simulink library "carnotUIBK"  (R2018b)
settings: Solver=VariableStepAuto  StartTime=0.0  StopTime=10.0  RelTol=1e-3  EnableMultiTasking=on
values from neighbouring files (symbols this model uses):
  A = 7*10*2    (= 140)    [theta_ground_v1.m]    (also in xlswrite1.m = num2cell(data))
  amb_factor = 1    [DOOR.m]    (also in WALL.m; WINDOW.m = 0)
  area = obj.width * obj.height    [DOOR.m]    (also in RES.m = []; ROOM.m = 0; THERMALZONE.m = area + room(kk).area; WALL.m = area - obj.doors(jj).calc_area())
  B = A/(0.5 * P)    (= 8.23529411765)    [theta_ground_v1.m]
  boundary = BOUNDARY()    [BUILDING.m]    (also in WALL.m = '')
  building = obj    [BUILDING.m]    (also in create_building_automatic.m = building.save(); ini_building_automatic.m = building.add_variant_hvac(building.variant_hvac, hvac); load_building_automatic.m = building.save())
  C = zeros(1,length(d)+1)    [CONSTRUCTION.m]    (also in DOOR.m = [0 0 0]; WALL.m = [0 0 0]; WINDOW.m = [0 0 0])
  control = 2    [GAIN.m]    (also in GAINS.m)
  cp = str2num(value)    [CONSTRUCTION.m]
  height = 0    [DOOR.m]    (also in ROOM.m; THERMALZONE.m; WALL.m; WINDOW.m)
  p = [timevec_weather weather(:,12)]    [BOUNDARY.m]    (also in WEATHER.m = 0; init_carnotUIBK.m = cell2mat(carnotUIBKpaths(i,2)))
  rho = str2num(value)    [CONSTRUCTION.m]    (also in theta_ground_v1.m = 2000)
  type = 1    [CONSTRUCTION.m]    (also in GAINS.m = raw_moisture{ii,3}; STRUCTURE.m = 0)
  view_factor = 1    [DOOR.m]    (also in WINDOW.m = 0)
  wall = []    [ROOM.m]
  z = obj.Z    [WALL.m]    (also in theta_ground_v1.m = 0)
  zone = obj.zone(ind)    [THERMALZONE.m]
undefined symbols (not defined in the file or in its folder): const, Dd, get_building, pos, Qdot_C, Qdot_H, Qdot_I_electricity, Qdot_I_light, Qdot_I_person, Qdot_S, Qdot_T_ground, Qdot_T_neighbour, Qdot_T_opaque, Qdot_T_window, Qdot_V_infiltration, Qdot_V_mech, Qdot_V_window, r_frame, solar_ratio, solar_ratio1, solar_ratio2, Tc, Tr, Ts, Uvalue, wallsurface, window, window_height, window_heigth, window_width, windowsurface, x_CO2, x_H2O, x_VOC
libraries: carnot x104, simulink x16, $bdroot x16, simulink_extras x14
(part 1 of 12)
settings Model: Creator=c8461199  LastModifiedBy=c8461246
settings DataIOCC: LimitDataPoints=on
settings OptimizationCC: LifeSpan=inf
settings DebuggingCC: AllowSymbolicDim=off  SFUnexpectedBacktrackingDiag=warning  SFNoUnconditionalDefaultTransitionDiag=warning  SFExecutionAtInitializationDiag=none
settings ModelReferenceCC: PropagateSignalLabelsOutOfModel=off
settings SFSimCC: SimUseLocalCustomCode=off
settings RTWCC: RTWUseLocalCustomCode=off
settings CodeAppCC: StateflowObjectComments=on
settings GRTTargetCC: TargetLangStandard=C89/C90 (ANSI)
settings ConfigComp: CovMetricSettings=dw  CovHtmlReporting=on  CovSaveCumulativeToWorkspaceVar=on  CovSaveSingleToWorkspaceVar=on  CovExternalEMLEnable=off

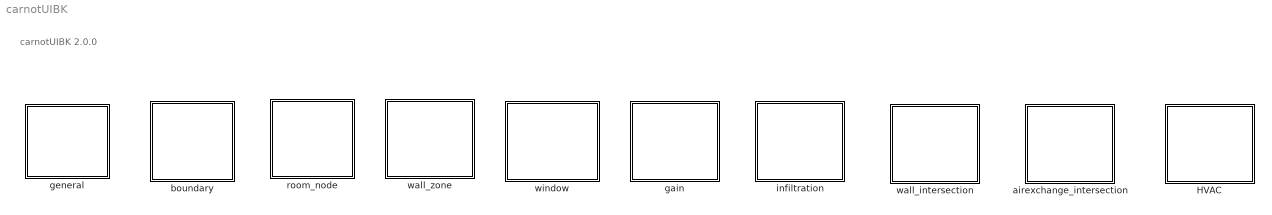
== system carnotUIBK ==
  note: carnotUIBK 2.0.0
  HVAC : Subsystem
  airexchange_intersection : Subsystem
  boundary : Subsystem
  gain : Subsystem
  general : Subsystem
  infiltration : Subsystem
  room_node : Subsystem
  wall_intersection : Subsystem
  wall_zone : Subsystem
  window : Subsystem

== system carnotUIBK/HVAC ==
  note: Group Definitions:
      |
      | Group 0: 	1 - 999		Internal use of carnotUIBK
      | Group 1000:	1001-1999	Heating Systems
      | Group 2000:	2001-2999	Ventilation Systems incl. air distribution
      |
      | Group 9000:	9001-9999	Control Systems
      |
      |
      |
      |
      | Please find the parameter sets in the folder 'HVAC_SYSTEM'!
  note: TEMPLATES
  note: Group 0: PHPP
  note: Group 1000: Heating Systems
  note: Group 2000: Ventilation Systems
  note: Group 9000: Control Systems
  HVAC_1001_electrical heaters : Subsystem  mask{building=get_building(building), system=1001}
      mask init:
      | hvac = building.hvac.get_system(system).parameter;
      mask Display: fprintf('%s \n(%d)',building.hvac.get_system(system).name,building.hvac.get_system(system).number)
  HVAC_1_PHPP : Subsystem  mask{building=get_building(building), system=1}
      mask init:
      | hvac = building.hvac.get_system(system).parameter;
      mask Display: fprintf('%s \n(%d)',building.hvac.get_system(system).name,building.hvac.get_system(system).number)
  HVAC_2001_ventilation system simple : Subsystem  mask{building=get_building(building), system=2001}
      mask init:
      | hvac = building.hvac.get_system(system).parameter;
      mask Display: fprintf('%s \n(%d)',building.hvac.get_system(system).name,building.hvac.get_system(system).number)
  HVAC_9001_window shading : Subsystem  mask{building=get_building(building), system=9001}
      mask init:
      | hvac = building.hvac.get_system(system).parameter;
      mask Display: fprintf('%s \n(%d)',building.hvac.get_system(system).name,building.hvac.get_system(system).number)
  HVAC_9002_window opening : Subsystem  mask{building=get_building(building), system=9002}
      mask init:
      | hvac = building.hvac.get_system(system).parameter;
      mask Display: fprintf('%s \n(%d)',building.hvac.get_system(system).name,building.hvac.get_system(system).number)
  HVAC_9003_door opening : Subsystem  mask{building=get_building(building), system=9003}
      mask init:
      | hvac = building.hvac.get_system(system).parameter;
      mask Display: fprintf('%s \n(%d)',building.hvac.get_system(system).name,building.hvac.get_system(system).number)
  HVAC_999_TEMPLATE : Subsystem  mask{building=get_building(building), system=[]}
      mask init:
      | hvac = building.hvac.get_system(system).parameter;
      mask Display: fprintf('%s \n(%d)',building.hvac.get_system(system).name,building.hvac.get_system(system).number)

== system carnotUIBK/airexchange_intersection ==
  EMPTY : Subsystem  VariantControl=(default)  mask(ACTIVE COMPONENT){}
      mask help:
      | This block represents the INFILTRATION from outdoors into a zone.
      | You can use this block also for window ventilation in one zone,
      | but you have to change the air_exchange_vector.
      |
      | [S] : vector for sinks and sources.
      |
      | NOTE: Mass flows of water and CO2 are taken into consideration.
      |
      | ASSUMPTION:
      | Incoming air volume flow is identical to outgoing air volume flow.
      mask Help: eval('man(''ventilation'')')
      mask Display:
      | plot([0.2 0.35], [0.8 0.7])
      | plot([0.35 0.65], [0.7 0.7])
      | plot([0.65 0.8], [0.7 0.8])
      | plot([0.65 0.8], [0.76 0.8])
      | plot([0.7 0.8], [0.65 0.8])
      | 
      | plot([0.2 0.35], [0.2 0.3])
      | plot([0.35 0.65], [0.3 0.3])
      | plot([0.65 0.8], [0.3 0.2])
      | plot([0.2 0.25], [0.2 0.32])
      | plot([0.2 0.35], [0.2 0.23])
      | 
      | plot ([0.45 0.45], [0 1])
      | plot ([0.55 0.55], [0 1])
      | 
      | plot ([0.45 0.55], [0.2 0.2])
      | plot ([0.45 0.55], [0.8 0.8])
      | 
      | plot ([0.45 0.55], [0 0.2])
      | plot ([0.45 0.55], [0.8 1])
  airexchange_empiric : Subsystem  VariantControl=V_i_1_2_inf1_m0  mask(ACTIVE COMPONENT){}
      mask help:
      | This block represents the INFILTRATION from outdoors into a zone.
      | You can use this block also for window ventilation in one zone,
      | but you have to change the air_exchange_vector.
      |
      | [S] : vector for sinks and sources.
      |
      | NOTE: Mass flows of water and CO2 are taken into consideration.
      |
      | ASSUMPTION:
      | Incoming air volume flow is identical to outgoing air volume flow.
      mask Help: eval('man(''ventilation'')')
      mask Display:
      | plot([0.2 0.35], [0.8 0.7])
      | plot([0.35 0.65], [0.7 0.7])
      | plot([0.65 0.8], [0.7 0.8])
      | plot([0.65 0.8], [0.76 0.8])
      | plot([0.7 0.8], [0.65 0.8])
      | 
      | plot([0.2 0.35], [0.2 0.3])
      | plot([0.35 0.65], [0.3 0.3])
      | plot([0.65 0.8], [0.3 0.2])
      | plot([0.2 0.25], [0.2 0.32])
      | plot([0.2 0.35], [0.2 0.23])
      | 
      | plot ([0.45 0.45], [0 1])
      | plot ([0.55 0.55], [0 1])
      | 
      | plot ([0.45 0.55], [0.2 0.2])
      | plot ([0.45 0.55], [0.8 0.8])
      | 
      | plot ([0.45 0.55], [0 0.2])
      | plot ([0.45 0.55], [0.8 1])
  airexchange_powerlaw : Subsystem  VariantControl=V_i_1_2_inf1_m1  mask(ACTIVE COMPONENT){}
      mask help:
      | This block represents the INFILTRATION from outdoors into a zone.
      | You can use this block also for window ventilation in one zone,
      | but you have to change the air_exchange_vector.
      |
      | [S] : vector for sinks and sources.
      |
      | NOTE: Mass flows of water and CO2 are taken into consideration.
      |
      | ASSUMPTION:
      | Incoming air volume flow is identical to outgoing air volume flow.
      mask Help: eval('man(''ventilation'')')
      mask Display:
      | plot([0.2 0.35], [0.8 0.7])
      | plot([0.35 0.65], [0.7 0.7])
      | plot([0.65 0.8], [0.7 0.8])
      | plot([0.65 0.8], [0.76 0.8])
      | plot([0.7 0.8], [0.65 0.8])
      | 
      | plot([0.2 0.35], [0.2 0.3])
      | plot([0.35 0.65], [0.3 0.3])
      | plot([0.65 0.8], [0.3 0.2])
      | plot([0.2 0.25], [0.2 0.32])
      | plot([0.2 0.35], [0.2 0.23])
      | 
      | plot ([0.45 0.45], [0 1])
      | plot ([0.55 0.55], [0 1])
      | 
      | plot ([0.45 0.55], [0.2 0.2])
      | plot ([0.45 0.55], [0.8 0.8])
      | 
      | plot ([0.45 0.55], [0 0.2])
      | plot ([0.45 0.55], [0.8 1])

== system carnotUIBK/boundary ==
  GDB : Subsystem  mask{building=get_building(building)}
      mask init:
      | b = building;
  NDB : Subsystem  mask{building=get_building(building)}
      mask init:
      | b = building;
  WDB : Subsystem  mask{building=get_building(building)}
      mask init:
      | we = building.boundary.weather;

== system carnotUIBK/gain ==
  EMPTY : Subsystem  VariantControl=(default)
  Equipment : Subsystem  VariantControl=V_z1_i1_m2
  Light : Subsystem  VariantControl=V_z1_i1_m1
  Moisture : Subsystem  VariantControl=V_z1_i1_m3
  People : Subsystem  VariantControl=V_z1_i1_m0

== system carnotUIBK/general ==
  AIB_initialize : $bdroot/room_node/EMPTY/AIB_initialize
  BDB_initialize : $bdroot/room_node/EMPTY/BDB_initialize
  S_initialize : Subsystem
  density and capacity : Subsystem
  x2RelHum_UIBK : carnot/Basic/Material_Properties/x2RelHum

== system carnotUIBK/infiltration ==
  EMPTY : Subsystem  VariantControl=(default)  mask(ACTIVE COMPONENT){}
      mask help:
      | This block represents the INFILTRATION from outdoors into a zone.
      | You can use this block also for window ventilation in one zone,
      | but you have to change the air_exchange_vector.
      |
      | [S] : vector for sinks and sources.
      |
      | NOTE: Mass flows of water and CO2 are taken into consideration.
      |
      | ASSUMPTION:
      | Incoming air volume flow is identical to outgoing air volume flow.
      mask Help: eval('man(''ventilation'')')
      mask Display:
      | plot([0.2 0.35], [0.8 0.7])
      | plot([0.35 0.65], [0.7 0.7])
      | plot([0.65 0.8], [0.7 0.8])
      | plot([0.65 0.8], [0.76 0.8])
      | plot([0.7 0.8], [0.65 0.8])
      | 
      | plot([0.2 0.35], [0.2 0.3])
      | plot([0.35 0.65], [0.3 0.3])
      | plot([0.65 0.8], [0.3 0.2])
      | plot([0.2 0.25], [0.2 0.32])
      | plot([0.2 0.35], [0.2 0.23])
      | 
      | plot ([0.45 0.45], [0 1])
      | plot ([0.55 0.55], [0 1])
      | 
      | plot ([0.45 0.55], [0.2 0.2])
      | plot ([0.45 0.55], [0.8 0.8])
      | 
      | plot ([0.45 0.55], [0 0.2])
      | plot ([0.45 0.55], [0.8 1])
  infiltration_constant : Subsystem  VariantControl=V_z1_inf1_m0  mask(ACTIVE COMPONENT){volume=z.heated_volume, n50=z.n50, wind_e=z.wind_e, co2=400}
      mask prompts: volume "heated volume"; wind_e "wind protection coefficent e"; co2 "CO2 content of air in ppm"
      mask help:
      | This block represents the INFILTRATION from outdoors into a zone.
      | You can use this block also for window ventilation in one zone,
      | but you have to change the air_exchange_vector.
      |
      | [S] : vector for sinks and sources.
      |
      | NOTE: Mass flows of water and CO2 are taken into consideration.
      |
      | ASSUMPTION:
      | Incoming air volume flow is identical to outgoing air volume flow.
      mask init:
      | CO2norm = co2*1e-6;
      | n_air = wind_e*n50;
      mask Help: eval('man(''ventilation'')')
      mask Display:
      | plot([0.2 0.35], [0.8 0.7])
      | plot([0.35 0.65], [0.7 0.7])
      | plot([0.65 0.8], [0.7 0.8])
      | plot([0.65 0.8], [0.76 0.8])
      | plot([0.7 0.8], [0.65 0.8])
      | 
      | plot([0.2 0.35], [0.2 0.3])
      | plot([0.35 0.65], [0.3 0.3])
      | plot([0.65 0.8], [0.3 0.2])
      | plot([0.2 0.25], [0.2 0.32])
      | plot([0.2 0.35], [0.2 0.23])
      | 
      | plot ([0.45 0.45], [0 1])
      | plot ([0.55 0.55], [0 1])
      | 
      | plot ([0.45 0.55], [0.2 0.2])
      | plot ([0.45 0.55], [0.8 0.8])
      | 
      | plot ([0.45 0.55], [0 0.2])
      | plot ([0.45 0.55], [0.8 1])
  infiltration_pressure : Subsystem  VariantControl=V_z1_inf1_m1  mask(ACTIVE COMPONENT){volume=z.heated_volume, n50=z.n50, wind_e=z.wind_e, co2=400}
      mask prompts: volume "heated volume"; wind_e "wind protection coefficent e"; co2 "CO2 content of air in ppm"
      mask help:
      | This block represents the INFILTRATION from outdoors into a zone.
      | You can use this block also for window ventilation in one zone,
      | but you have to change the air_exchange_vector.
      |
      | [S] : vector for sinks and sources.
      |
      | NOTE: Mass flows of water and CO2 are taken into consideration.
      |
      | ASSUMPTION:
      | Incoming air volume flow is identical to outgoing air volume flow.
      mask init:
      | CO2norm = co2*1e-6;
      | n_air = wind_e*n50;
      mask Help: eval('man(''ventilation'')')
      mask Display:
      | plot([0.2 0.35], [0.8 0.7])
      | plot([0.35 0.65], [0.7 0.7])
      | plot([0.65 0.8], [0.7 0.8])
      | plot([0.65 0.8], [0.76 0.8])
      | plot([0.7 0.8], [0.65 0.8])
      | 
      | plot([0.2 0.35], [0.2 0.3])
      | plot([0.35 0.65], [0.3 0.3])
      | plot([0.65 0.8], [0.3 0.2])
      | plot([0.2 0.25], [0.2 0.32])
      | plot([0.2 0.35], [0.2 0.23])
      | 
      | plot ([0.45 0.45], [0 1])
      | plot ([0.55 0.55], [0 1])
      | 
      | plot ([0.45 0.55], [0.2 0.2])
      | plot ([0.45 0.55], [0.8 0.8])
      | 
      | plot ([0.45 0.55], [0 0.2])
      | plot ([0.45 0.55], [0.8 1])

== system carnotUIBK/room_node ==
  1-node : Subsystem  VariantControl=V_z1_m2  mask(NODE){zoneairvolume=z.heated_volume, zoneheight=z.heated_volume/z.heated_area, zonestartTEMP=z.t_ini, zonestartWATER=z.phi_ini, zonestartCO2=z.CO2_ini, zonestartVOC=z.VOC_ini, zonestartP0=1e5/(293.15)*(273.15+z.t_ini), timeconst=z.timeconstant, mcp=z.cp_spec*z.heated_area}
      mask prompts: zoneairvolume "SIZE: netto air volume >0, m^3"; zoneheight "SIZE: height of zone (floor - ceiling) >0, m"; zonestartTEMP "START TEMPERATURE: convective and radiative node, °C"; zonestartWATER "START AIR HUMIDITY: relative air humidity [0,100], %"; zonestartCO2 "START CO2: start value CO2, ppm"; zonestartVOC "START VOC:"; zonestartP0 "START P0:"; timeconst "timeconstant of radiative and convective node in s"; mcp "cp_spec*area"
      mask help: This subsystem represents the variant for a 1-NODE room node.
      mask init:
      | %CO2norm = 400*10^-6;
      | zoneairvolume = max(0.01, zoneairvolume);
      | zoneheight = max(0.01, zoneheight);
      | zonestartWATER = min(100, max(0, zonestartWATER));
      | zonestartWATER = rel_hum2x(zonestartTEMP, 10^5, zonestartWATER)*1.18*zoneairvolume; % kg H2O in zone volume (at 20°C)
      | 
      | zonestartCO2 = zonestartCO2*10^-6*1.529*zoneairvolume; % kg CO2 in zone volume
      | zonestartAIR = 10^5*zoneairvolume/(287*(zonestartTEMP+273)); % kg AIR in zone volume
      mask Help: web(fullfile(path_carnot('help'),'Room_Node.html'),'-helpbrowser')
  1-node_womass : Subsystem  VariantControl=V_z1_m4  mask(NODE){zoneairvolume=z.heated_volume, zoneheight=z.heated_volume/z.heated_area, zonestartTEMP=z.t_ini, zonestartWATER=z.phi_ini, zonestartCO2=z.CO2_ini, zonestartVOC=z.VOC_ini, zonestartP0=1e5/(293.15)*(273.15+z.t_ini), timeconst=z.timeconstant, mcp=z.cp_spec*z.heated_area}
      mask prompts: zoneairvolume "SIZE: netto air volume >0, m^3"; zoneheight "SIZE: height of zone (floor - ceiling) >0, m"; zonestartTEMP "START TEMPERATURE: convective and radiative node, °C"; zonestartWATER "START AIR HUMIDITY: relative air humidity [0,100], %"; zonestartCO2 "START CO2: start value CO2, ppm"; zonestartVOC "START VOC:"; zonestartP0 "START P0:"; timeconst "timeconstant of radiative and convective node in s"; mcp "cp_spec*area"
      mask help:
      | This NOCE- block delivers the energy consumption, temperature and air quality of a zone.
      | It is assumed that this node represents the center of a zone all connected sink and source blocks communicate with. Sink and source blocks are walls, windows, persons, heater etc..
      |
      | [S] : input vector from sink blocks and source blocks
      | [AIV] : output vector with node temperature and air quality data.
      mask init: same as carnotUIBK/room_node/1-node
      mask Help: web(fullfile(path_carnot('help'),'Room_Node.html'),'-helpbrowser')
  2-node : Subsystem  VariantControl=V_z1_m3  mask(NODE){zoneairvolume=z.heated_volume, zoneheight=z.heated_volume/z.heated_area, zonestartTEMP=z.t_ini, zonestartWATER=z.phi_ini, zonestartCO2=z.CO2_ini, zonestartVOC=z.VOC_ini, zonestartP0=1e5/(293.15)*(273.15+z.t_ini), timeconst=z.timeconstant}
      mask prompts: zoneairvolume "SIZE: netto air volume >0, m^3"; zoneheight "SIZE: height of zone (floor - ceiling) >0, m"; zonestartTEMP "START TEMPERATURE: convective and radiative node, °C"; zonestartWATER "START AIR HUMIDITY: relative air humidity [0,100], %"; zonestartCO2 "START CO2: start value CO2, ppm"; zonestartVOC "START VOC:"; zonestartP0 "START P0:"; timeconst "timeconstant of radiative and convective node in s"
      mask help: This subsystem represents the variant for a 2-NODE room node.
      mask init:
      | %CO2norm = 400*10^-6;
      | zoneairvolume = max(0.01, zoneairvolume);
      | zoneheight = max(0.01, zoneheight);
      | zonestartWATER = min(100, max(0, zonestartWATER));
      | zonestartWATER = rel_hum2x(zonestartTEMP, 10^5, zonestartWATER)*1.18*zoneairvolume; % kg H2O in zone volume (at 20°C)
      | 
      | zonestartCO2 = zonestartCO2*10^-6*1.529*zoneairvolume; % kg CO2 in zone volume
      | zonestartAIR = 1e5*zoneairvolume/(287*(zonestartTEMP+273.15)); % kg AIR in zone volume
      | %zonestartAIR = 9.5e4*zoneairvolume/(287*(zonestartTEMP+273.15)); % kg AIR in zone volume
      mask Help: web(fullfile(path_carnot('help'),'Room_Node.html'),'-helpbrowser')
  2-node_ideal : Subsystem  VariantControl=V_z1_m1  mask(NODE){zoneairvolume=z.heated_volume, zoneheight=z.heated_volume/z.heated_area, zonestartTEMP=z.t_ini, zonestartWATER=z.phi_ini, zonestartCO2=z.CO2_ini, zonestartVOC=z.VOC_ini, zonestartP0=1e5/(293.15)*(273.15+z.t_ini), timeconst=z.timeconstant, temperature_timevalues=z.profile_timevalues, temperature_timeduration=z.profile_timeduration, temperature_Tc=z.profile_Tc, temperature_Tr=z.profile_Tc}
      mask prompts: zoneairvolume "SIZE: netto air volume >0, m^3"; zoneheight "SIZE: height of zone (floor - ceiling) >0, m"; zonestartTEMP "START TEMPERATURE: convective and radiative node, °C"; zonestartWATER "START AIR HUMIDITY: relative air humidity [0,100], %"; zonestartCO2 "START CO2: start value CO2, ppm"; zonestartVOC "START VOC:"; zonestartP0 "START P0:"; timeconst "timeconstant of radiative and convective node in s"
      mask help: This subsystem represents the variant for a 2-NODE room node with IDEAL HEATING.
      mask init: same as carnotUIBK/room_node/1-node
      mask Help: web(fullfile(path_carnot('help'),'Room_Node.html'),'-helpbrowser')
  EMPTY : Subsystem  VariantControl=(default)  mask(NODE){temperature_timevalues=z.profile_timevalues, temperature_timeduration=z.profile_timeduration, temperature_Tc=z.profile_Tc, temperature_Tr=z.profile_Tr, temperature_rH=z.profile_rH, temperature_CO2=z.profile_CO2, temperature_VOC=z.profile_VOC, temperature_p=z.profile_p}
      mask help: This subsystem represents the variant for an EMPTY room node.
      mask Help: web(fullfile(path_carnot('help'),'Room_Node.html'),'-helpbrowser')

== system carnotUIBK/wall_intersection ==
  EMPTY : Subsystem  VariantControl=(default)
      mask help: This subsystem represents the variant for an EMPTY wall type.
  R-C model : Subsystem  VariantControl=V_i_1_2_w1_m1  mask{t0=z.t_ini, d=fliplr(const.parameter.xmesh_beu), cond=fliplr(const.parameter.lambda), cwall=fliplr(const.parameter.cp), rho=fliplr(const.parameter.rho), reflectground=0.2, abs_emiss=[const.absorption_2 const.emission_2 const.emission_1], tau=const.parameter.tau, dactive=const.parameter.d_active}
      mask prompts: t0 "initial temperature [degree centigrade]"; d "thickness of nodes [m] (vector)"; cond "conductivity of nodes [W/(m*K)] (vector)"; cwall "capacity of nodes [J/(kg*K)] (vector)"; rho "density [kg/m^3]"; reflectground "reflection of ground"; abs_emiss "[outer absorption, outer emission, inner emisson]"; tau "time-constant of wall [s]"; dactive "depth of active layer in m from outside (-1, if none)"
      mask help: This subsystem represents the variant for an R-C wall type.
      mask init:
      | absorption_out = min(1, max(abs_emiss(1),0));
      | nodes = length(d);
      | emission_in = abs_emiss(3);
      | emission_out = abs_emiss(2);
      | active = 0;
      | if (dactive>=0) active=1; end
      | 
      | %für Variablen in shaderad
      | %wallangle = pos(1);
      | %wallazimut = pos(2);
      | %wallheight = h;
      | %wallwidth = w;
  UA : Subsystem  VariantControl=V_i_1_2_w1_m0  mask{U=const.parameter.U}
      mask prompts: U "U-value without he and hi [W/(m^2*K]]"
      mask help: This subsystem represents the variant for an UA wall type.
  hygrothermal model : Subsystem  VariantControl=V_i_1_2_w1_m2  mask{t0=z.t_ini, reflectground=0.2, abs_emiss=[const.absorption_2 const.emission_2 const.emission_1], xmesh=const.parameter.xmesh_hygro, X=const.parameter.X, d=const.parameter.d, lambda=const.parameter.lambda_hygro, rho=const.parameter.rho_hygro, cp=const.parameter.cp_hygro, mu=const.parameter.mu, ufs=const.parameter.ufs, FSF_u=const.parameter.FSF_u, FSF_phi=const.parameter.FSF_phi, FSF_dudphi=const.parameter.FSF_dudphi, FSF_k=const.parameter.FSF_k, K_kleff=const.parameter.K_kleff, K_u=const.parameter.K_u, K_kl=const.parameter.K_kl, FSF_length=const.parameter.FSF_length, K_length=const.parameter.K_length, T_ini=const.parameter.T_ini_hygro, Phi_ini=const.parameter.Phi_ini_hygro, T_source=const.parameter.T_source, Phi_source=const.parameter.Phi_source, Tdactive=const.parameter.T_dactive, Phidactive=const.parameter.Phi_dactive}
      mask prompts: t0 "initial temperature [degree centigrade]"; reflectground "reflection of ground"; abs_emiss "[outer absorption, outer emission, inner emisson]"
      mask help: This subsystem represents the variant for an HYGROTHERMAL wall type.
      mask init:
      | absorption_out = min(1, max(abs_emiss(1),0));
      | nodes = length(d);
      | emission_in = abs_emiss(3);
      | emission_out = abs_emiss(2);

== system carnotUIBK/wall_zone ==
  EMPTY : Subsystem  VariantControl=(default)
      mask help: This subsystem represents the variant for an EMPTY wall type.
  R-C model : Subsystem  VariantControl=V_z1_w1_m1  mask{t0=z.t_ini, d=fliplr(const.parameter.xmesh_beu), cond=fliplr(const.parameter.lambda), cwall=fliplr(const.parameter.cp), rho=fliplr(const.parameter.rho), reflectground=0.2, abs_emiss=[const.absorption_2 const.emission_2 const.emission_1], tau=const.parameter.tau, dactive=const.parameter.d_active}
      mask prompts: t0 "initial temperature [degree centigrade]"; d "thickness of nodes [m] (vector)"; cond "conductivity of nodes [W/(m*K)] (vector)"; cwall "capacity of nodes [J/(kg*K)] (vector)"; rho "density [kg/m^3]"; reflectground "reflection of ground"; abs_emiss "[outer absorption, outer emission, inner emisson]"; tau "time-constant of wall [s]"; dactive "depth of active layer in m from outside (-1, if none)"
      mask help: This subsystem represents the variant for an R-C wall type.
      mask init:
      | absorption_out = min(1, max(abs_emiss(1),0));
      | nodes = length(d);
      | emission_in = abs_emiss(3);
      | emission_out = abs_emiss(2);
      | active = 0;
      | if (dactive>=0) active=1; end
      | 
      | %für Variablen in shaderad
      | %wallangle = pos(1);
      | %wallazimut = pos(2);
      | %wallheight = h;
      | %wallwidth = w;
      | nodes = length(d);
  UA : Subsystem  VariantControl=V_z1_w1_m0  mask{U=const.parameter.U}
      mask prompts: U "U-value without he and hi [W/(m^2*K]]"
      mask help: This subsystem represents the variant for an UA wall type.
  hygrothermal model : Subsystem  VariantControl=V_z1_w1_m2  mask{t0=z.t_ini, reflectground=0.2, abs_emiss=[const.absorption_2 const.emission_2 const.emission_1], xmesh=const.parameter.xmesh_hygro, X=const.parameter.X, d=const.parameter.d, lambda=const.parameter.lambda_hygro, rho=const.parameter.rho_hygro, cp=const.parameter.cp_hygro, mu=const.parameter.mu, ufs=const.parameter.ufs, FSF_u=const.parameter.FSF_u, FSF_phi=const.parameter.FSF_phi, FSF_dudphi=const.parameter.FSF_dudphi, FSF_k=const.parameter.FSF_k, K_kleff=const.parameter.K_kleff, K_u=const.parameter.K_u, K_kl=const.parameter.K_kl, FSF_length=const.parameter.FSF_length, K_length=const.parameter.K_length, T_ini=const.parameter.T_ini_hygro, Phi_ini=const.parameter.Phi_ini_hygro, T_source=const.parameter.T_source, Phi_source=const.parameter.Phi_source, Tdactive=const.parameter.T_dactive, Phidactive=const.parameter.Phi_dactive}
      mask prompts: t0 "initial temperature [degree centigrade]"; reflectground "reflection of ground"; abs_emiss "[outer absorption, outer emission, inner emisson]"
      mask help: This subsystem represents the variant for an HYGROTHERMAL wall type.
      mask init:
      | absorption_out = min(1, max(abs_emiss(1),0));
      | nodes = length(d);
      | emission_in = abs_emiss(3);
      | emission_out = abs_emiss(2);

== system carnotUIBK/window ==
  note: FORGET THIS STUPID MODEL!!!!
  EMTPY : Subsystem  VariantControl=(default)  mask(window){}
      mask help:
      | The window model evaluates the g-value, the total energy transmission tau and the u-value to build up a two node model.
      |
      | control [0..1]:   specifies the fraction of the shading device.
      |                   0 means a norm g-value, 1 means total shading of the
      |                   window
      mask Help: web(fullfile(path_carnot('help'),'Window.html'),'-helpbrowser')
  window_CARNOT : Subsystem  VariantControl=V_z1_wi1_m1  mask(outer wall){wallsize=[window_heigth window_width], frame=r_frame, pos=pos, t0=z.t_ini, d=const.parameter.d_w, cond=const.parameter.lambda_w, cwall=const.parameter.c_w, rho=const.parameter.rho_w, misc=[0.20 const.absorption_2 const.emission_2 const.emission_1], gvalue=const.parameter.g_w, dactive=[0.01 0.05]}
      mask prompts: wallsize "size of window [m] [height width]"; frame "part of frame of the surface (0..1)"; pos "azimut (0=south, east = -90)"; t0 "initial temperature [degree centigrade]"; d "thickness of nodes [m] (vector)"; cond "conductivity of nodes [W/(m*K)] (vector)"; cwall "capacity of nodes [J/(kg*K)] (vector)"; rho "density [kg/m^3]"; misc "[reflection_ground absorption_out emission_out emission_in]"; gvalue "energy transmission of window (0..1)"; dactive "depth of active layer [m] (-1, if none; start at outside)"
      mask help:
      | This is the model of a window of a house.
      | first element of the vector = layer to surrounding
      | last element of the vector = layer to room
      |
      | control [0..1]:   specifies the fraction of the shading device.
      |                   0 means a norm g-value, 1 means total shading of the
      |                   window
      mask init:
      | nodes = length(d);
      | numlayer = nodes;
      | 
      | h = wallsize(1);
      | w = wallsize(2);
      | %für Variablen in shaderad
      | reflectground = min(0, max(1, misc(1)));
      | 
      | wallangle = position(1);
      | wallazimut = position(2);
      | wallheight=h;
      | wallwidth=w;
      | wallsurface = h*w;
      | 
      | for i = 1:numpanes
      |     C = sum(cwall(i)*d(i)*d(i)*rho(i));
      | end
      | R = 1/Ug-(0.04+0.13);
      | tau = R*C/2;
      | 
      | absorption_out = misc(2);
      | emission_out = misc(3);
      | emission_in = misc(4);
      mask Help: web(fullfile(path_carnot('help'),'Window.html'),'-helpbrowser')
  window_TF : Subsystem  VariantControl=V_z1_wi1_m0  mask(window){windowsize=[window_heigth window_width], numpanes=const.parameter.n_pane, frame=r_frame, pos=pos, d=const.parameter.d_w, rho=const.parameter.rho_w, cp=const.parameter.c_w, t0=z.t_ini, misc=[0.20 const.absorption_2 const.emission_2 const.emission_1], gvalue=const.parameter.g_w, tauzero=const.parameter.tau_g_w, Ug=Uvalue, shad_type=No shading, type_glazing=Dreifach-Wärmeschutzglas, tau_shad=0.304, bli_a=0.08, bli_b=0.0126, bli_c=0.009, bli_d=0.062, bli_alpha=45, bli_refl=0.441}
      mask prompts: windowsize "size of window [m] [height width]"; numpanes "number of window panes [1..4]"; frame "part of frame of the surface (0..1)"; pos "azimut (0=south, east = -90)"; d "thickness of panes [m]"; rho "density of glass [kg/m³]"; cp "capacity of glass [J/(kgK)]"; t0 "initial temperature [degree centigrade]"; misc "[reflection_ground absorption_out emission_out emission_in]"; gvalue "energy transmission of window (g-value) [0..1]"; tauzero "transmission of glass [0..1]"; Ug "heat transfer coefficient (U-value) [W/m²K]"; shad_type "shading type [no Shading/exterior/interior]"; type_glazing "glazing type"; tau_shad "solar transmittance of shading element [0..1]"; bli_a "a  Depth of blind blades [m]"; bli_b "b heigth of blind blades [m]"; bli_c "c distance of "b" to back end of blind blade [m]"; bli_d "d offset between blind blades [m]"; bli_alpha "blind angle  (0=closed, 90=horizontal) [0..90]"; bli_refl "optical reflectance of blind surface [0..1]"
      mask help:
      | The window model evaluates the g-value, the total energy transmission tau and the u-value to build up a two node model.
      |
      | control [0..1]:   specifies the fraction of the shading device.
      |                   0 means a norm g-value, 1 means total shading of the
      |                   window
      mask init:
      | h = windowsize(1);
      | w = windowsize(2);
      | 
      | reflectground = max(0, min(1, misc(1)));
      | windowsurface = h*w;
      | 
      | absorption_out = misc(2);
      | emission_out = misc(3);
      | emission_in = misc(4);
      | 
      | for i = 1:numpanes
      |     C = sum(cp(i)*d(i)*d(i)*rho(i));
      | end
      | R = 1/Ug-(0.04+0.13);
      | timeconst = R*C/2;
      | 
      | R_norm_in = 0.13;
      | R_norm_out = 0.04;
      | Rwin = 1/Ug - R_norm_in - R_norm_out;
      mask Help: web(fullfile(path_carnot('help'),'Window.html'),'-helpbrowser')
      mask TypeOptions shad_type: No shading | Exterior Screen | Interior Screen | Venetian Blind
      mask Callback shad_type:
      | switch get_param(gcb,'shad_type')
      |         case 'No shading' % nr. 1 no shading
      |             set_param(gcb,'MaskVisibilities',{'on','on','on','on','on','on','on','on','on','on','on','on','on','off','off','off','off','off','off','off','off'});
      |         case 'Exterior Screen' % nr. 2 external screen
      |             set_param(gcb,'MaskVisibilities',{'on','on','on','on','on','on','on','on','on','on','on','on','on','off','on','off','off','off','off','off','off'});
      |         case 'Interior Screen' % nr. 3 Interior Screen
      |             set_param(gcb,'MaskVisibilities',{'on','on','on','on','on','on','on','on','on','on','on','on','on','on','on','off','off','off','off','off','off'});
      |         case 'Venetian Blind' % nr. 4 venetian blind
      |             set_param(gcb,'MaskVisibilities',{'on','on','on','on','on','on','on','on','on','on','on','on','on','off','off','on','on','on','on','on','on'});
      |     end
      mask TypeOptions type_glazing: Zweifachglas normal | Zweifach-Wärmeschutzglas | Zweifach-Kombiglas 73/41 | Zweifach-Kombiglas 50/24 | Dreifachglas normal | Dreifach-Wärmeschutzglas
  window_TF_shading : Subsystem  VariantControl=V_z1_wi1_m2  mask(window){windowsize=[window_heigth window_width], numpanes=const.parameter.n_pane, frame=r_frame, pos=pos, d=const.parameter.d_w, rho=const.parameter.rho_w, cp=const.parameter.c_w, t0=z.t_ini, misc=[0.20 const.absorption_2 const.emission_2 const.emission_1], gvalue=const.parameter.g_w, tauzero=const.parameter.tau_g_w, Ug=Uvalue, shad_type=Exterior Screen, type_glazing=Dreifach-Wärmeschutzglas, tau_shad=const.parameter.solar_transmittance, bli_a=const.parameter.venetianblind_a, bli_b=const.parameter.venetianblind_b, bli_c=const.parameter.venetianblind_c, bli_d=const.parameter.venetianblind_d, bli_alpha=const.parameter.venetianblind_angle, bli_refl=const.parameter.venetianblind_reflect}
      mask prompts: windowsize "size of window [m] [height width]"; numpanes "number of window panes [1..4]"; frame "part of frame of the surface (0..1)"; pos "azimut (0=south, east = -90)"; d "thickness of panes [m]"; rho "density of glass [kg/m³]"; cp "capacity of glass [J/(kgK)]"; t0 "initial temperature [degree centigrade]"; misc "[reflection_ground absorption_out emission_out emission_in]"; gvalue "energy transmission of window (g-value) [0..1]"; tauzero "transmission of glass [0..1]"; Ug "heat transfer coefficient (U-value) [W/m²K]"; shad_type "shading type [no Shading/exterior/interior]"; type_glazing "glazing type"; tau_shad "solar transmittance of shading element [0..1]"; bli_a "a  Depth of blind blades [m]"; bli_b "b heigth of blind blades [m]"; bli_c "c distance of "b" to back end of blind blade [m]"; bli_d "d offset between blind blades [m]"; bli_alpha "blind angle  (0=closed, 90=horizontal) [0..90]"; bli_refl "optical reflectance of blind surface [0..1]"
      mask help:
      | The window model evaluates the g-value, the total energy transmission tau and the u-value to build up a two node model.
      |
      | control [0..1]:   specifies the fraction of the shading device.
      |                   0 means a norm g-value, 1 means total shading of the
      |                   window
      mask init: same as carnotUIBK/window/window_TF
      mask Help: web(fullfile(path_carnot('help'),'Window.html'),'-helpbrowser')
      mask TypeOptions shad_type: No shading | Exterior Screen | Interior Screen | Venetian Blind
      mask Callback shad_type:
      | switch get_param(gcb,'shad_type')
      |         case 'No shading' % nr. 1 no shading
      |             set_param(gcb,'MaskVisibilities',{'on','on','on','on','on','on','on','on','on','on','on','on','on','off','off','off','off','off','off','off','off'});
      |         case 'Exterior Screen' % nr. 2 external screen
      |             set_param(gcb,'MaskVisibilities',{'on','on','on','on','on','on','on','on','on','on','on','on','on','off','on','off','off','off','off','off','off'});
      |         case 'Interior Screen' % nr. 3 Interior Screen
      |             set_param(gcb,'MaskVisibilities',{'on','on','on','on','on','on','on','on','on','on','on','on','on','on','on','off','off','off','off','off','off'});
      |         case 'Venetian Blind' % nr. 4 venetian blind
      |             set_param(gcb,'MaskVisibilities',{'on','on','on','on','on','on','on','on','on','on','on','on','on','off','off','on','on','on','on','on','on'});
      |     end
      mask TypeOptions type_glazing: Zweifachglas normal | Zweifach-Wärmeschutzglas | Zweifach-Kombiglas 73/41 | Zweifach-Kombiglas 50/24 | Dreifachglas normal | Dreifach-Wärmeschutzglas

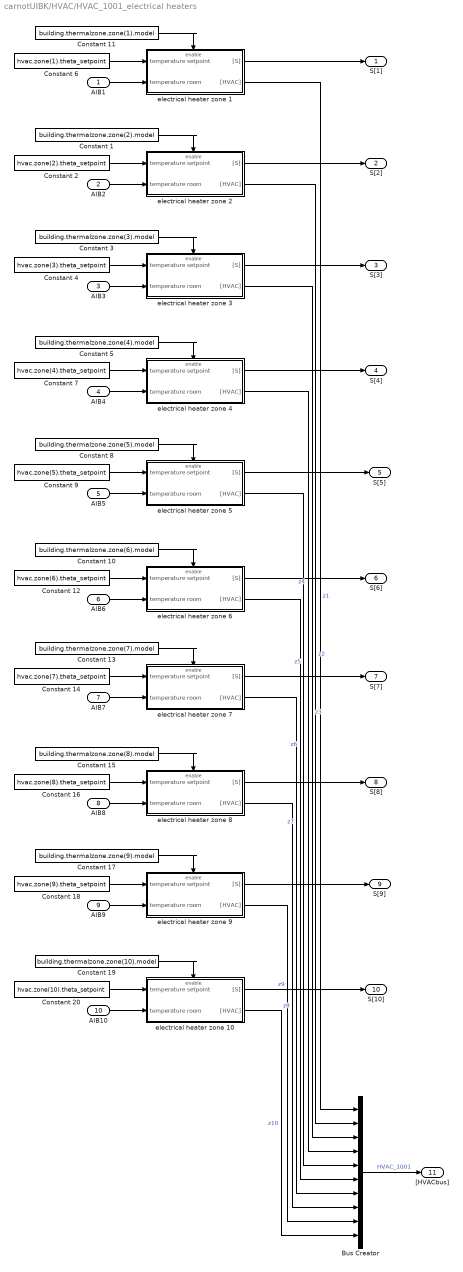
== system carnotUIBK/HVAC/HVAC_1001_electrical heaters ==
  AIB1 : Inport
  AIB2 : Inport  Port=2
  AIB3 : Inport  Port=3
  AIB4 : Inport  Port=4
  AIB5 : Inport  Port=5
  AIB6 : Inport  Port=6
  AIB7 : Inport  Port=7
  AIB8 : Inport  Port=8
  AIB9 : Inport  Port=9
  AIB10 : Inport  Port=10
  Bus Creator : BusCreator  Inputs=10
  Constant 1 : Constant  Value=building.thermalzone.zone(2).model  VectorParams1D=off
  Constant 10 : Constant  Value=building.thermalzone.zone(6).model  VectorParams1D=off
  Constant 11 : Constant  Value=building.thermalzone.zone(1).model  VectorParams1D=off
  Constant 12 : Constant  Value=hvac.zone(6).theta_setpoint  VectorParams1D=off
  Constant 13 : Constant  Value=building.thermalzone.zone(7).model  VectorParams1D=off
  Constant 14 : Constant  Value=hvac.zone(7).theta_setpoint  VectorParams1D=off
  Constant 15 : Constant  Value=building.thermalzone.zone(8).model  VectorParams1D=off
  Constant 16 : Constant  Value=hvac.zone(8).theta_setpoint  VectorParams1D=off
  Constant 17 : Constant  Value=building.thermalzone.zone(9).model  VectorParams1D=off
  Constant 18 : Constant  Value=hvac.zone(9).theta_setpoint  VectorParams1D=off
  Constant 19 : Constant  Value=building.thermalzone.zone(10).model  VectorParams1D=off
  Constant 2 : Constant  Value=hvac.zone(2).theta_setpoint  VectorParams1D=off
  Constant 20 : Constant  Value=hvac.zone(10).theta_setpoint  VectorParams1D=off
  Constant 3 : Constant  Value=building.thermalzone.zone(3).model  VectorParams1D=off
  Constant 4 : Constant  Value=hvac.zone(3).theta_setpoint  VectorParams1D=off
  Constant 5 : Constant  Value=building.thermalzone.zone(4).model  VectorParams1D=off
  Constant 6 : Constant  Value=hvac.zone(1).theta_setpoint  VectorParams1D=off
  Constant 7 : Constant  Value=hvac.zone(4).theta_setpoint  VectorParams1D=off
  Constant 8 : Constant  Value=building.thermalzone.zone(5).model  VectorParams1D=off
  Constant 9 : Constant  Value=hvac.zone(5).theta_setpoint  VectorParams1D=off
  electrical heater zone 1 : Subsystem  mask{max_power=hvac.zone(1).max_power, timeconst=hvac.zone(1).timeconst, s_conv=hvac.zone(1).s_conv, Kp=hvac.zone(1).Kp, Tn=hvac.zone(1).Tn}
      mask prompts: max_power "maximal power"; timeconst "timeconstant radiator"; s_conv "share to convective node"; Kp "PI controller: Kp"; Tn "PI controller: Tn"
  electrical heater zone 10 : Subsystem  mask{max_power=hvac.zone(10).max_power, timeconst=hvac.zone(10).timeconst, s_conv=hvac.zone(10).s_conv, Kp=hvac.zone(10).Kp, Tn=hvac.zone(10).Tn}
      mask prompts: max_power "maximal power"; timeconst "timeconstant radiator"; s_conv "share to convective node"; Kp "PI controller: Kp"; Tn "PI controller: Tn"
  electrical heater zone 2 : Subsystem  mask{max_power=hvac.zone(2).max_power, timeconst=hvac.zone(2).timeconst, s_conv=hvac.zone(2).s_conv, Kp=hvac.zone(2).Kp, Tn=hvac.zone(2).Tn}
      mask prompts: max_power "maximal power"; timeconst "timeconstant radiator"; s_conv "share to convective node"; Kp "PI controller: Kp"; Tn "PI controller: Tn"
  electrical heater zone 3 : Subsystem  mask{max_power=hvac.zone(3).max_power, timeconst=hvac.zone(3).timeconst, s_conv=hvac.zone(3).s_conv, Kp=hvac.zone(3).Kp, Tn=hvac.zone(3).Tn}
      mask prompts: max_power "maximal power"; timeconst "timeconstant radiator"; s_conv "share to convective node"; Kp "PI controller: Kp"; Tn "PI controller: Tn"
  electrical heater zone 4 : Subsystem  mask{max_power=hvac.zone(4).max_power, timeconst=hvac.zone(4).timeconst, s_conv=hvac.zone(4).s_conv, Kp=hvac.zone(4).Kp, Tn=hvac.zone(4).Tn}
      mask prompts: max_power "maximal power"; timeconst "timeconstant radiator"; s_conv "share to convective node"; Kp "PI controller: Kp"; Tn "PI controller: Tn"
  electrical heater zone 5 : Subsystem  mask{max_power=hvac.zone(5).max_power, timeconst=hvac.zone(5).timeconst, s_conv=hvac.zone(5).s_conv, Kp=hvac.zone(5).Kp, Tn=hvac.zone(5).Tn}
      mask prompts: max_power "maximal power"; timeconst "timeconstant radiator"; s_conv "share to convective node"; Kp "PI controller: Kp"; Tn "PI controller: Tn"
  electrical heater zone 6 : Subsystem  mask{max_power=hvac.zone(6).max_power, timeconst=hvac.zone(6).timeconst, s_conv=hvac.zone(6).s_conv, Kp=hvac.zone(6).Kp, Tn=hvac.zone(6).Tn}
      mask prompts: max_power "maximal power"; timeconst "timeconstant radiator"; s_conv "share to convective node"; Kp "PI controller: Kp"; Tn "PI controller: Tn"
  electrical heater zone 7 : Subsystem  mask{max_power=hvac.zone(7).max_power, timeconst=hvac.zone(7).timeconst, s_conv=hvac.zone(7).s_conv, Kp=hvac.zone(7).Kp, Tn=hvac.zone(7).Tn}
      mask prompts: max_power "maximal power"; timeconst "timeconstant radiator"; s_conv "share to convective node"; Kp "PI controller: Kp"; Tn "PI controller: Tn"
  electrical heater zone 8 : Subsystem  mask{max_power=hvac.zone(8).max_power, timeconst=hvac.zone(8).timeconst, s_conv=hvac.zone(8).s_conv, Kp=hvac.zone(8).Kp, Tn=hvac.zone(8).Tn}
      mask prompts: max_power "maximal power"; timeconst "timeconstant radiator"; s_conv "share to convective node"; Kp "PI controller: Kp"; Tn "PI controller: Tn"
  electrical heater zone 9 : Subsystem  mask{max_power=hvac.zone(9).max_power, timeconst=hvac.zone(9).timeconst, s_conv=hvac.zone(9).s_conv, Kp=hvac.zone(9).Kp, Tn=hvac.zone(9).Tn}
      mask prompts: max_power "maximal power"; timeconst "timeconstant radiator"; s_conv "share to convective node"; Kp "PI controller: Kp"; Tn "PI controller: Tn"
  S[1] : Outport
  S[2] : Outport  Port=2
  S[3] : Outport  Port=3
  S[4] : Outport  Port=4
  S[5] : Outport  Port=5
  S[6] : Outport  Port=6
  S[7] : Outport  Port=7
  S[8] : Outport  Port=8
  S[9] : Outport  Port=9
  S[10] : Outport  Port=10
  "[HVACbus]" : Outport  Port=11  InitialOutput=0
  wires:
  AIB1/1 -> electrical heater zone 1/2(temperature room)
  electrical heater zone 1/1("[S]") -> S[1]/1
  Constant 11/1 -> electrical heater zone 1/Enable
  Constant 6/1 -> electrical heater zone 1/1(temperature setpoint)
  Constant 2/1 -> electrical heater zone 2/1(temperature setpoint)
  Constant 1/1 -> electrical heater zone 2/Enable
  AIB2/1 -> electrical heater zone 2/2(temperature room)
  Constant 3/1 -> electrical heater zone 3/Enable
  Constant 4/1 -> electrical heater zone 3/1(temperature setpoint)
  Constant 7/1 -> electrical heater zone 4/1(temperature setpoint)
  Constant 5/1 -> electrical heater zone 4/Enable
  Constant 8/1 -> electrical heater zone 5/Enable
  Constant 9/1 -> electrical heater zone 5/1(temperature setpoint)
  Constant 12/1 -> electrical heater zone 6/1(temperature setpoint)
  Constant 10/1 -> electrical heater zone 6/Enable
  Constant 13/1 -> electrical heater zone 7/Enable
  Constant 14/1 -> electrical heater zone 7/1(temperature setpoint)
  Constant 16/1 -> electrical heater zone 8/1(temperature setpoint)
  Constant 15/1 -> electrical heater zone 8/Enable
  Constant 17/1 -> electrical heater zone 9/Enable
  Constant 18/1 -> electrical heater zone 9/1(temperature setpoint)
  Constant 20/1 -> electrical heater zone 10/1(temperature setpoint)
  Constant 19/1 -> electrical heater zone 10/Enable
  AIB10/1 -> electrical heater zone 10/2(temperature room)
  AIB9/1 -> electrical heater zone 9/2(temperature room)
  AIB8/1 -> electrical heater zone 8/2(temperature room)
  AIB7/1 -> electrical heater zone 7/2(temperature room)
  AIB5/1 -> electrical heater zone 5/2(temperature room)
  AIB6/1 -> electrical heater zone 6/2(temperature room)
  AIB4/1 -> electrical heater zone 4/2(temperature room)
  AIB3/1 -> electrical heater zone 3/2(temperature room)
  Bus Creator/1 -> "[HVACbus]"/1  "HVAC_1001"
  electrical heater zone 2/1("[S]") -> S[2]/1
  electrical heater zone 3/1("[S]") -> S[3]/1
  electrical heater zone 4/1("[S]") -> S[4]/1
  electrical heater zone 5/1("[S]") -> S[5]/1
  electrical heater zone 6/1("[S]") -> S[6]/1
  electrical heater zone 7/1("[S]") -> S[7]/1
  electrical heater zone 8/1("[S]") -> S[8]/1
  electrical heater zone 9/1("[S]") -> S[9]/1
  electrical heater zone 10/1("[S]") -> S[10]/1
  electrical heater zone 1/2("[HVAC]") -> Bus Creator/1  "z1"
  electrical heater zone 2/2("[HVAC]") -> Bus Creator/2  "z2"
  electrical heater zone 3/2("[HVAC]") -> Bus Creator/3  "z3"
  electrical heater zone 4/2("[HVAC]") -> Bus Creator/4  "z4"
  electrical heater zone 5/2("[HVAC]") -> Bus Creator/5  "z5"
  electrical heater zone 6/2("[HVAC]") -> Bus Creator/6  "z6"
  electrical heater zone 7/2("[HVAC]") -> Bus Creator/7  "z7"
  electrical heater zone 8/2("[HVAC]") -> Bus Creator/8  "z8"
  electrical heater zone 9/2("[HVAC]") -> Bus Creator/9  "z9"
  electrical heater zone 10/2("[HVAC]") -> Bus Creator/10  "z10"
